simulink model "GPCA_CONFIG"  (Simulink 8.7)
settings: Solver=FixedStepDiscrete  StartTime=0.0  StopTime=10.0  RelTol=1e-3
libraries: simulink x1
settings Model: Creator=bourbouh  LastModifiedBy=bourbouh
settings DataIOCC: LimitDataPoints=off  SaveFormat=Dataset
settings DebuggingCC: UnderspecifiedInitializationDetection=Simplified  MergeDetectMultiDrivingBlocksExec=error
settings HardwareCC: ProdBitPerPointer=64  ProdLargestAtomicFloat=Float  ProdIntDivRoundTo=Zero  ProdEndianess=LittleEndian  ProdWordSize=64  ProdHWDeviceType=Intel->x86-64 (Windows64)
settings ModelReferenceCC: PropagateSignalLabelsOutOfModel=on
settings ConfigComp: CovModelRefEnable=off

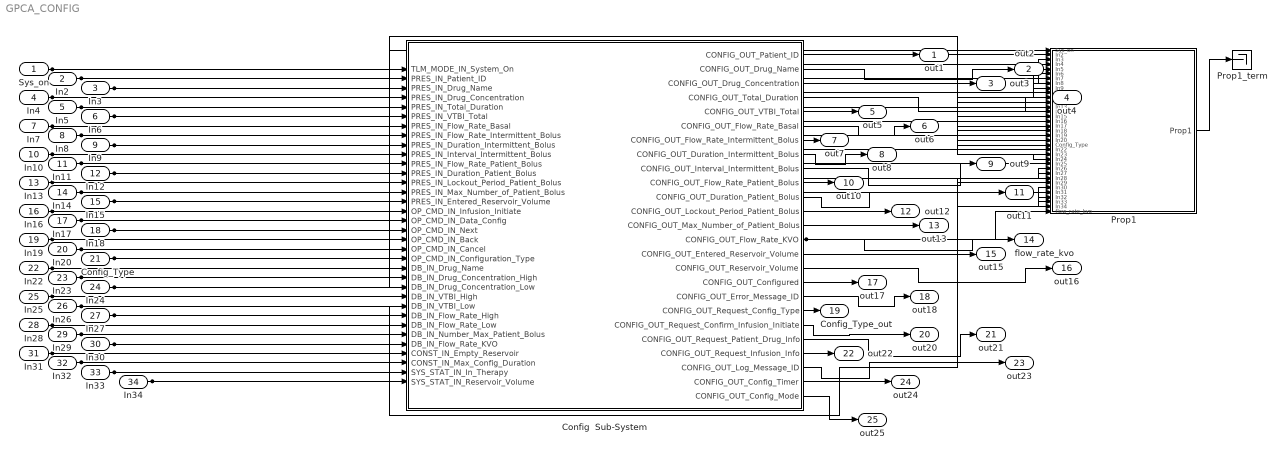
== system GPCA_CONFIG ==
  Sys_on : Inport
  In2 : Inport  Port=2
  In3 : Inport  Port=3
  In4 : Inport  Port=4
  In5 : Inport  Port=5
  In6 : Inport  Port=6
  In7 : Inport  Port=7
  In8 : Inport  Port=8
  In9 : Inport  Port=9
  In10 : Inport  Port=10
  In11 : Inport  Port=11
  In12 : Inport  Port=12
  In13 : Inport  Port=13
  In14 : Inport  Port=14
  In15 : Inport  Port=15
  In16 : Inport  Port=16
  In17 : Inport  Port=17
  In18 : Inport  Port=18
  In19 : Inport  Port=19
  In20 : Inport  Port=20
  Config_Type : Inport  Port=21
  In22 : Inport  Port=22
  In23 : Inport  Port=23
  In24 : Inport  Port=24
  In25 : Inport  Port=25
  In26 : Inport  Port=26
  In27 : Inport  Port=27
  In28 : Inport  Port=28
  In29 : Inport  Port=29
  In30 : Inport  Port=30
  In31 : Inport  Port=31
  In32 : Inport  Port=32
  In33 : Inport  Port=33
  In34 : Inport  Port=34
  Config  Sub-System : Stateflow chart  TreatAsAtomicUnit=on
  Prop1 : Subsystem  TreatAsAtomicUnit=on  mask(Observer){AnnotationType=ensures, ObserverType=[]}
      mask prompts: AnnotationType "Type of annotation (pre/post...)"; ObserverType "Observer type"
      mask help:
      | Set an observer for the system.
      | The annotation type parameter sets the type of observer:
      | - requires : pre-condition
      | - ensures : post-condition
      | - assert : an assertion
      | - observer : the observer computes a special type of properties
      mask TypeOptions AnnotationType: ensures | requires | assert | observer
      mask Callback AnnotationType:
      | paramStr = get_param(gcb, 'MaskValues');
      | if strcmp(paramStr{1}(1),'o')
      | set_param(gcb,'MaskVisibilities',{'on';'on'});
      | paramStr{2} = 'ellipsoid';
      | set_param(gcb,'MaskValues',paramStr);
      | else
      | set_param(gcb,'MaskVisibilities',{'on';'off'});
      | end
      | clear paramStr;
      mask Callback ObserverType:
      | paramStr = get_param(gcb, 'MaskValues');
      | if strcmp(paramStr{1}(1),'o')
      | set_param(gcb,'MaskVisibilities',{'on';'on'});
      | paramStr{2} = 'ellipsoid';
      | set_param(gcb,'MaskValues',paramStr);
      | else
      | set_param(gcb,'MaskVisibilities',{'on';'off'});
      | end
      | clear paramStr;
      mask Display:
      | color('black')
      | text(0.5, 0.5, ['Property: ''' get_param(gcb,'name') ''''], 'horizontalAlignment', 'center');
      | text(0.99, 0.03, '{\bf\fontsize{12}CEX}', 'hor', 'right', 'ver', 'bottom', 'texmode', 'on');
  Prop1_term : Terminator
  out1 : Outport
  out2 : Outport  Port=2
  out3 : Outport  Port=3
  out4 : Outport  Port=4
  out5 : Outport  Port=5
  out6 : Outport  Port=6
  out7 : Outport  Port=7
  out8 : Outport  Port=8
  out9 : Outport  Port=9
  out10 : Outport  Port=10
  out11 : Outport  Port=11
  out12 : Outport  Port=12
  out13 : Outport  Port=13
  flow_rate_kvo : Outport  Port=14
  out15 : Outport  Port=15
  out16 : Outport  Port=16
  out17 : Outport  Port=17
  out18 : Outport  Port=18
  Config_Type_out : Outport  Port=19
  out20 : Outport  Port=20
  out21 : Outport  Port=21
  out22 : Outport  Port=22
  out23 : Outport  Port=23
  out24 : Outport  Port=24
  out25 : Outport  Port=25
  wires:
  Config  Sub-System/2(CONFIG_OUT_Drug_Name) -> out2/1
  Config  Sub-System/3(CONFIG_OUT_Drug_Concentration) -> out3/1
  Config  Sub-System/1(CONFIG_OUT_Patient_ID) -> out1/1
  Config  Sub-System/4(CONFIG_OUT_Total_Duration) -> out4/1
  Config  Sub-System/5(CONFIG_OUT_VTBI_Total) -> out5/1
  Config  Sub-System/6(CONFIG_OUT_Flow_Rate_Basal) -> out6/1
  Config  Sub-System/7(CONFIG_OUT_Flow_Rate_Intermittent_Bolus) -> out7/1
  Config  Sub-System/8(CONFIG_OUT_Duration_Intermittent_Bolus) -> out8/1
  Config  Sub-System/9(CONFIG_OUT_Interval_Intermittent_Bolus) -> out9/1
  Config  Sub-System/12(CONFIG_OUT_Lockout_Period_Patient_Bolus) -> out12/1
  Config  Sub-System/10(CONFIG_OUT_Flow_Rate_Patient_Bolus) -> out10/1
  Config  Sub-System/11(CONFIG_OUT_Duration_Patient_Bolus) -> out11/1
  Config  Sub-System/14(CONFIG_OUT_Flow_Rate_KVO) -> flow_rate_kvo/1, Prop1/35(flow_rate_kvo)
  Config  Sub-System/15(CONFIG_OUT_Entered_Reservoir_Volume) -> out15/1
  Config  Sub-System/13(CONFIG_OUT_Max_Number_of_Patient_Bolus) -> out13/1
  Config  Sub-System/16(CONFIG_OUT_Reservoir_Volume) -> out16/1
  Config  Sub-System/17(CONFIG_OUT_Configured) -> out17/1
  Config  Sub-System/18(CONFIG_OUT_Error_Message_ID) -> out18/1
  Config  Sub-System/20(CONFIG_OUT_Request_Confirm_Infusion_Initiate) -> out20/1
  Config  Sub-System/21(CONFIG_OUT_Request_Patient_Drug_Info) -> out21/1
  Config  Sub-System/24(CONFIG_OUT_Config_Timer) -> out24/1
  Config  Sub-System/22(CONFIG_OUT_Request_Infusion_Info) -> out22/1
  Config  Sub-System/23(CONFIG_OUT_Log_Message_ID) -> out23/1
  Config  Sub-System/19(CONFIG_OUT_Request_Config_Type) -> Config_Type_out/1
  Config  Sub-System/25(CONFIG_OUT_Config_Mode) -> out25/1
  Sys_on/1 -> Config  Sub-System/1(TLM_MODE_IN_System_On), Prop1/1(Sys_on)
  In2/1 -> Config  Sub-System/2(PRES_IN_Patient_ID), Prop1/2(In2)
  In3/1 -> Config  Sub-System/3(PRES_IN_Drug_Name), Prop1/3(In3)
  In4/1 -> Config  Sub-System/4(PRES_IN_Drug_Concentration), Prop1/4(In4)
  In5/1 -> Config  Sub-System/5(PRES_IN_Total_Duration), Prop1/5(In5)
  In6/1 -> Config  Sub-System/6(PRES_IN_VTBI_Total), Prop1/6(In6)
  In7/1 -> Config  Sub-System/7(PRES_IN_Flow_Rate_Basal), Prop1/7(In7)
  In8/1 -> Config  Sub-System/8(PRES_IN_Flow_Rate_Intermittent_Bolus), Prop1/8(In8)
  In9/1 -> Config  Sub-System/9(PRES_IN_Duration_Intermittent_Bolus), Prop1/9(In9)
  In10/1 -> Config  Sub-System/10(PRES_IN_Interval_Intermittent_Bolus), Prop1/10(In10)
  In11/1 -> Config  Sub-System/11(PRES_IN_Flow_Rate_Patient_Bolus), Prop1/11(In11)
  In12/1 -> Config  Sub-System/12(PRES_IN_Duration_Patient_Bolus), Prop1/12(In12)
  In13/1 -> Config  Sub-System/13(PRES_IN_Lockout_Period_Patient_Bolus), Prop1/13(In13)
  In14/1 -> Config  Sub-System/14(PRES_IN_Max_Number_of_Patient_Bolus), Prop1/14(In14)
  In15/1 -> Config  Sub-System/15(PRES_IN_Entered_Reservoir_Volume), Prop1/15(In15)
  In16/1 -> Config  Sub-System/16(OP_CMD_IN_Infusion_Initiate), Prop1/16(In16)
  In17/1 -> Config  Sub-System/17(OP_CMD_IN_Data_Config), Prop1/17(In17)
  In18/1 -> Config  Sub-System/18(OP_CMD_IN_Next), Prop1/18(In18)
  In19/1 -> Config  Sub-System/19(OP_CMD_IN_Back), Prop1/19(In19)
  In20/1 -> Config  Sub-System/20(OP_CMD_IN_Cancel), Prop1/20(In20)
  Config_Type/1 -> Config  Sub-System/21(OP_CMD_IN_Configuration_Type), Prop1/21(Config_Type)
  In22/1 -> Config  Sub-System/22(DB_IN_Drug_Name), Prop1/22(In22)
  In23/1 -> Config  Sub-System/23(DB_IN_Drug_Concentration_High), Prop1/23(In23)
  In24/1 -> Config  Sub-System/24(DB_IN_Drug_Concentration_Low), Prop1/24(In24)
  In25/1 -> Config  Sub-System/25(DB_IN_VTBI_High), Prop1/25(In25)
  In26/1 -> Config  Sub-System/26(DB_IN_VTBI_Low), Prop1/26(In26)
  In27/1 -> Config  Sub-System/27(DB_IN_Flow_Rate_High), Prop1/27(In27)
  In28/1 -> Config  Sub-System/28(DB_IN_Flow_Rate_Low), Prop1/28(In28)
  In29/1 -> Config  Sub-System/29(DB_IN_Number_Max_Patient_Bolus), Prop1/29(In29)
  In30/1 -> Config  Sub-System/30(DB_IN_Flow_Rate_KVO), Prop1/30(In30)
  In31/1 -> Config  Sub-System/31(CONST_IN_Empty_Reservoir), Prop1/31(In31)
  In32/1 -> Config  Sub-System/32(CONST_IN_Max_Config_Duration), Prop1/32(In32)
  In33/1 -> Config  Sub-System/33(SYS_STAT_IN_In_Therapy), Prop1/33(In33)
  In34/1 -> Config  Sub-System/34(SYS_STAT_IN_Reservoir_Volume), Prop1/34(In34)
  Prop1/1(Prop1) -> Prop1_term/1

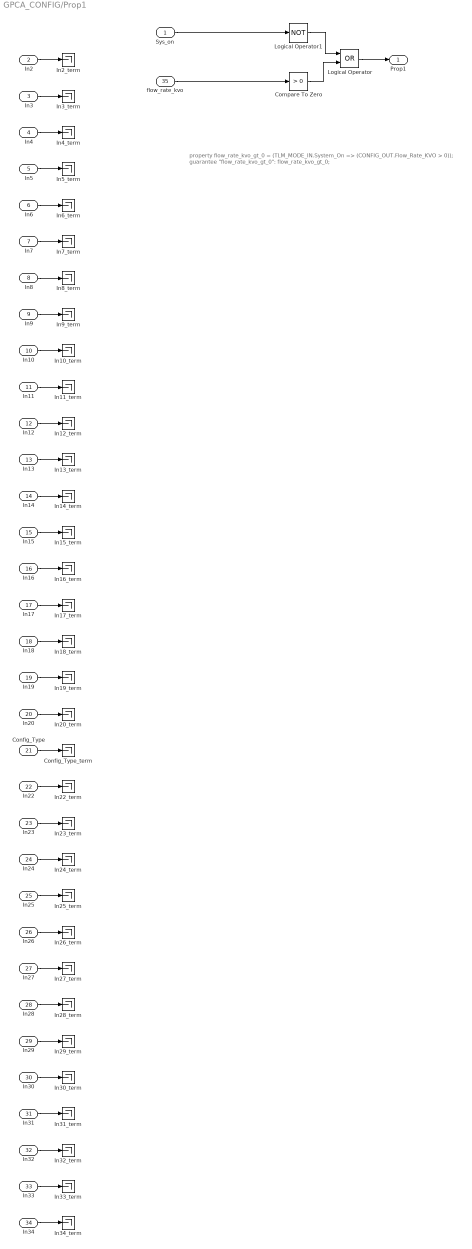
== system GPCA_CONFIG/Prop1 ==
  note: property flow_rate_kvo_gt_0 =
      | (TLM_MODE_IN.System_On => (CONFIG_OUT.Flow_Rate_KVO > 0));
      |
      | guarantee "flow_rate_kvo_gt_0": flow_rate_kvo_gt_0;
  Sys_on : Inport
  In2 : Inport  Port=2
  In3 : Inport  Port=3
  In4 : Inport  Port=4
  In5 : Inport  Port=5
  In6 : Inport  Port=6
  In7 : Inport  Port=7
  In8 : Inport  Port=8
  In9 : Inport  Port=9
  In10 : Inport  Port=10
  In11 : Inport  Port=11
  In12 : Inport  Port=12
  In13 : Inport  Port=13
  In14 : Inport  Port=14
  In15 : Inport  Port=15
  In16 : Inport  Port=16
  In17 : Inport  Port=17
  In18 : Inport  Port=18
  In19 : Inport  Port=19
  In20 : Inport  Port=20
  Config_Type : Inport  Port=21
  In22 : Inport  Port=22
  In23 : Inport  Port=23
  In24 : Inport  Port=24
  In25 : Inport  Port=25
  In26 : Inport  Port=26
  In27 : Inport  Port=27
  In28 : Inport  Port=28
  In29 : Inport  Port=29
  In30 : Inport  Port=30
  In31 : Inport  Port=31
  In32 : Inport  Port=32
  In33 : Inport  Port=33
  In34 : Inport  Port=34
  flow_rate_kvo : Inport  Port=35
  Compare To Zero : simulink/Logic and Bit Operations/Compare To Zero  relop=>  OutDataTypeStr=boolean
  Config_Type_term : Terminator
  In10_term : Terminator
  In11_term : Terminator
  In12_term : Terminator
  In13_term : Terminator
  In14_term : Terminator
  In15_term : Terminator
  In16_term : Terminator
  In17_term : Terminator
  In18_term : Terminator
  In19_term : Terminator
  In20_term : Terminator
  In22_term : Terminator
  In23_term : Terminator
  In24_term : Terminator
  In25_term : Terminator
  In26_term : Terminator
  In27_term : Terminator
  In28_term : Terminator
  In29_term : Terminator
  In2_term : Terminator
  In30_term : Terminator
  In31_term : Terminator
  In32_term : Terminator
  In33_term : Terminator
  In34_term : Terminator
  In3_term : Terminator
  In4_term : Terminator
  In5_term : Terminator
  In6_term : Terminator
  In7_term : Terminator
  In8_term : Terminator
  In9_term : Terminator
  Logical Operator : Logic  Operator=OR  AllPortsSameDT=off  OutDataTypeStr=boolean
  Logical Operator1 : Logic  Operator=NOT  AllPortsSameDT=off  OutDataTypeStr=boolean
  Prop1 : Outport
  wires:
  Sys_on/1 -> Logical Operator1/1
  In2/1 -> In2_term/1
  In3/1 -> In3_term/1
  In4/1 -> In4_term/1
  In5/1 -> In5_term/1
  In6/1 -> In6_term/1
  In7/1 -> In7_term/1
  In8/1 -> In8_term/1
  In9/1 -> In9_term/1
  In10/1 -> In10_term/1
  In11/1 -> In11_term/1
  In12/1 -> In12_term/1
  In13/1 -> In13_term/1
  In14/1 -> In14_term/1
  In15/1 -> In15_term/1
  In16/1 -> In16_term/1
  In17/1 -> In17_term/1
  In18/1 -> In18_term/1
  In19/1 -> In19_term/1
  In20/1 -> In20_term/1
  Config_Type/1 -> Config_Type_term/1
  In22/1 -> In22_term/1
  In23/1 -> In23_term/1
  In24/1 -> In24_term/1
  In25/1 -> In25_term/1
  In26/1 -> In26_term/1
  In27/1 -> In27_term/1
  In28/1 -> In28_term/1
  In29/1 -> In29_term/1
  In30/1 -> In30_term/1
  In31/1 -> In31_term/1
  In32/1 -> In32_term/1
  In33/1 -> In33_term/1
  In34/1 -> In34_term/1
  flow_rate_kvo/1 -> Compare To Zero/1
  Logical Operator/1 -> Prop1/1
  Logical Operator1/1 -> Logical Operator/1
  Compare To Zero/1 -> Logical Operator/2

== stateflow chart Config  Sub-System ==
  state Configuration
    state Prescription_Config
      entry: CONFIG_OUT_Config_Timer++;
      CONFIG_OUT_Reservoir_Volume=SYS_STAT_IN_Reservoir_Volume;
      CONFIG_OUT_Config_Mode=2;
      checkIfPrescriptionAvailable();
      during: CONFIG_OUT_Config_Timer++;
      CONFIG_OUT_Reservoir_Volume=SYS_STAT_IN_Reservoir_Volume;
      checkIfPrescriptionAvailable();
      exit: CONFIG_OUT_Config_Timer++;
      state Patient_Drug_info
        entry: CONFIG_OUT_Config_Mode=3;
        during: CONFIG_OUT_Config_Mode=3;
        exit: CONFIG_OUT_Config_Mode=3;
        state GetParam
          entry:t_PatientID=PRES_IN_Patient_ID;
          t_DrugName=PRES_IN_Drug_Name;
          t_DrugConcentration=PRES_IN_Drug_Concentration;
          t_EnteredReservoirVolume = PRES_IN_Entered_Reservoir_Volume;
          CONFIG_OUT_Request_Patient_Drug_Info=0;
        state DisplayParam
          entry:CONFIG_OUT_Request_Patient_Drug_Info=1;
          validate=0;
        state GetDrugSafeValues
          entry:CONFIG_OUT_Drug_Name=t_DrugName;
          value = CheckDrugName(t_DrugName, DB_IN_Drug_Name);
          during:value = CheckDrugName(t_DrugName, DB_IN_Drug_Name);
        state DisplayErrorMessage
          entry:CONFIG_OUT_Error_Message_ID=5;
        state ValidateParam
          entry:validate= checkPatient_DrugParam(t_DrugConcentration, DB_IN_Drug_Concentration_Low, DB_IN_Drug_Concentration_High, t_EnteredReservoirVolume, CONST_IN_Empty_Reservoir);
          CONFIG_OUT_Request_Patient_Drug_Info=0;
          value=0;
          during:validate= checkPatient_DrugParam(t_DrugConcentration, DB_IN_Drug_Concentration_Low, DB_IN_Drug_Concentration_High, t_EnteredReservoirVolume, CONST_IN_Empty_Reservoir);
          CONFIG_OUT_Request_Patient_Drug_Info=0;
          value=0;
        state v= checkPatient_DrugParam(t_DrugConcentration, DB_IN_Drug_Concentration_Low, DB_IN_Drug_Concentration_High, t_EnteredReservoirVolume, CONST_IN_Empty_Reservoir) [function]
          (default) -> (junction 59) : {v=1;}
          (junction 59) -> (junction 60) [order 1] : [t_DrugConcentration < DB_IN_Drug_Concentration_Low || t_DrugConcentration > DB_IN_Drug_Concentration_High ] {v=0;}
          (junction 59) -> (junction 61) [order 2] : [t_EnteredReservoirVolume < CONST_IN_Empty_Reservoir] {v=0;}
        state y= CheckDrugName(z, DB_IN_Drug_Name) [function]
          (default) -> (junction 68) : {y=1;}
          (junction 68) -> (junction 69) : [z != DB_IN_Drug_Name] {y=0;}
        DisplayParam -> GetParam [order 1] : [OP_CMD_IN_Next == 1]
        (default) -> DisplayParam
        DisplayParam -> ValidateParam [order 2] : [OP_CMD_IN_Next == 1]
        DisplayErrorMessage -> DisplayParam
        GetParam -> GetDrugSafeValues : [OP_CMD_IN_Next == 1]{value=0;}
        GetDrugSafeValues -> DisplayErrorMessage [order 2] : [value==0]
        ValidateParam -> DisplayErrorMessage [order 1] : [validate==0]
        GetDrugSafeValues -> ValidateParam [order 1] : [value==1]
      state SelectType
        entry:CONFIG_OUT_Request_Config_Type=1;
      state Infusion_info
        entry: CONFIG_OUT_Config_Mode=4;
        during: CONFIG_OUT_Config_Mode=4;
        exit: CONFIG_OUT_Config_Mode=4;
        state GetInfusionParam
          entry:t_VTBI_total =PRES_IN_VTBI_Total;
          t_Duration_total =PRES_IN_Total_Duration;
          t_FlowRate_basal =PRES_IN_Flow_Rate_Basal;
          t_FlowRate_sbolus = PRES_IN_Flow_Rate_Intermittent_Bolus;
          t_FlowRate_pbolus =PRES_IN_Flow_Rate_Patient_Bolus;
          t_Duration_sbolus =PRES_IN_Duration_Intermittent_Bolus;
          t_Duration_pbolus =PRES_IN_Duration_Patient_Bolus;
          t_LockOutPeriod_pbolus=PRES_IN_Lockout_Period_Patient_Bolus;
          t_NumberMax_pbolus =PRES_IN_Max_Number_of_Patient_Bolus;
          t_Interval_sbolus =PRES_IN_Interval_Intermittent_Bolus;
          t_FlowRate_kvo =DB_IN_Flow_Rate_KVO;
          CONFIG_OUT_Request_Infusion_Info=0;
        state RequestInfusionParam
          entry :CONFIG_OUT_Request_Infusion_Info=1;
          validate=0;
        state ValidateInfusionParam
          entry: checkInfusionParam();
          during: checkInfusionParam();
        state checkInfusionParam [function]
          (default) -> (junction 79) : {validate=1;}
          (junction 79) -> (junction 78) [order 1] : [t_VTBI_total > DB_IN_VTBI_High || t_VTBI_total < DB_IN_VTBI_Low]{validate=0;}
          (junction 79) -> (junction 80) [order 2] : [t_FlowRate_basal < DB_IN_Flow_Rate_Low || t_FlowRate_basal > DB_IN_Flow_Rate_High]{validate=0;}
          (junction 79) -> (junction 81) [order 3] : [t_FlowRate_sbolus < DB_IN_Flow_Rate_Low || t_FlowRate_sbolus > DB_IN_Flow_Rate_High]{validate=0;}
          (junction 79) -> (junction 82) [order 4] : [t_FlowRate_pbolus< DB_IN_Flow_Rate_Low || t_FlowRate_pbolus > DB_IN_Flow_Rate_High]{validate=0;}
          (junction 79) -> (junction 83) [order 5] : [t_Duration_sbolus  > t_Interval_sbolus]{validate=0;}
          (junction 79) -> (junction 85) [order 7] : [t_FlowRate_pbolus < t_FlowRate_basal || t_FlowRate_sbolus < t_FlowRate_basal ]{validate=0;}
          (junction 79) -> (junction 84) [order 6] : [t_NumberMax_pbolus >  DB_IN_Number_Max_Patient_Bolus]{validate=0;}
        RequestInfusionParam -> GetInfusionParam [order 1] : [OP_CMD_IN_Next == 1]
        (default) -> RequestInfusionParam
        ValidateInfusionParam -> RequestInfusionParam [order 1] : [validate==0]
        RequestInfusionParam -> ValidateInfusionParam [order 2] : [OP_CMD_IN_Next == 1]
        GetInfusionParam -> ValidateInfusionParam : [OP_CMD_IN_Next == 1]
      state ConfirmInfusionInitation
        entry:CONFIG_OUT_Request_Confirm_Infusion_Initiate = 1;
        during: CONFIG_OUT_Request_Confirm_Infusion_Initiate = 1;
      (default) -> SelectType
      SelectType -> (junction 34) : [OP_CMD_IN_Configuration_Type>0] {CONFIG_OUT_Request_Config_Type=0;Selected_Configuration_Type=OP_CMD_IN_Configuration_Type;copyCurrentValuesToTemp();}
      (junction 34) -> Patient_Drug_info [order 2]
      (junction 34) -> Infusion_info [order 1] : [SYS_STAT_IN_In_Therapy]
      Infusion_info -> Patient_Drug_info : [OP_CMD_IN_Back && !SYS_STAT_IN_In_Therapy]
      ValidateParam -> Infusion_info [order 2] : [validate==1]
      ValidateInfusionParam -> ConfirmInfusionInitation [order 2] : [validate==1]
    state MAIN
      entry: CONFIG_OUT_Config_Mode=1;
      CONFIG_OUT_Config_Timer=0;
      setReservoirVolume();
      checkIfPrescriptionAvailable();
      during: CONFIG_OUT_Config_Mode=1;
      CONFIG_OUT_Config_Timer=0;
      setReservoirVolume();
      checkIfPrescriptionAvailable();
      exit: CONFIG_OUT_Config_Mode=1;
      CONFIG_OUT_Config_Timer=0;
      setReservoirVolume();
      checkIfPrescriptionAvailable();
    state copyCurrentValuesToTemp [function]
      (default) -> (junction 94) : {t_PatientID= CONFIG_OUT_Patient_ID;
          | t_DrugName=CONFIG_OUT_Drug_Name;
          | t_DrugConcentration= CONFIG_OUT_Drug_Concentration;
          | t_EnteredReservoirVolume=CONFIG_OUT_Entered_Reservoir_Volume;
          | t_VTBI_total=CONFIG_OUT_VTBI_Total;
          | t_Duration_total=CONFIG_OUT_Total_Duration;
          | t_FlowRate_basal=CONFIG_OUT_Flow_Rate_Basal;
          | t_FlowRate_sbolus=CONFIG_OUT_Flow_Rate_Intermittent_Bolus;
          | t_FlowRate_pbolus=CONFIG_OUT_Flow_Rate_Patient_Bolus;
          | t_FlowRate_kvo=CONFIG_OUT_Flow_Rate_KVO;
          | t_Duration_sbolus=CONFIG_OUT_Duration_Intermittent_Bolus;
          | t_Duration_pbolus=CONFIG_OUT_Duration_Patient_Bolus;
          | t_LockOutPeriod_pbolus=CONFIG_OUT_Lockout_Period_Patient_Bolus;
          | t_NumberMax_pbolus=CONFIG_OUT_Max_Number_of_Patient_Bolus;
          | t_Interval_sbolus=CONFIG_OUT_Interval_Intermittent_Bolus;
          | t_EnteredReservoirVolume=CONFIG_OUT_Entered_Reservoir_Volume;}
    state saveConfigValues [function]
      (default) -> (junction 96) : {CONFIG_OUT_Patient_ID=t_PatientID;
          | CONFIG_OUT_Drug_Name=t_DrugName;
          | CONFIG_OUT_Drug_Concentration=t_DrugConcentration;
          | CONFIG_OUT_Entered_Reservoir_Volume = t_EnteredReservoirVolume;
          | CONFIG_OUT_VTBI_Total =t_VTBI_total;
          | CONFIG_OUT_Total_Duration =t_Duration_total;
          | CONFIG_OUT_Flow_Rate_Basal =t_FlowRate_basal;
          | CONFIG_OUT_Flow_Rate_Intermittent_Bolus = t_FlowRate_sbolus;
          | CONFIG_OUT_Flow_Rate_Patient_Bolus =t_FlowRate_pbolus;
          | CONFIG_OUT_Flow_Rate_KVO =t_FlowRate_kvo;
          | CONFIG_OUT_Duration_Intermittent_Bolus =t_Duration_sbolus;
          | CONFIG_OUT_Duration_Patient_Bolus =t_Duration_pbolus;
          | CONFIG_OUT_Lockout_Period_Patient_Bolus =t_LockOutPeriod_pbolus;
          | CONFIG_OUT_Max_Number_of_Patient_Bolus =t_NumberMax_pbolus;
          | CONFIG_OUT_Interval_Intermittent_Bolus =t_Interval_sbolus;
          | CONFIG_OUT_Reservoir_Volume=CONFIG_OUT_Entered_Reservoir_Volume;
          | CONFIG_OUT_Configured=Selected_Configuration_Type;
          | New_Configuration=1;
          | /*cancelConfigValues();*/
          | /*comment it because it is in the same level*/
          | /*Try to call cancelConfigValues every time you call the current function*/
          | writeLog(1);}
    state cancelConfigValues [function]
      (default) -> (junction 98) : {t_PatientID=0;
          | t_DrugName=0;
          | t_DrugConcentration=0;
          | t_EnteredReservoirVolume =0;
          | t_VTBI_total =0 ;
          | t_Duration_total =0 ;
          | t_FlowRate_basal =0 ;
          | t_FlowRate_sbolus =0 ;
          | t_FlowRate_pbolus =0 ;
          | t_FlowRate_kvo =0 ;
          | t_Duration_sbolus =0 ;
          | t_Duration_pbolus =0 ;
          | t_LockOutPeriod_pbolus =0 ;
          | t_NumberMax_pbolus =0 ;
          | t_Interval_sbolus =0 ;
          | writeLog(2);}
    state checkIfPrescriptionAvailable [function]
      (default) -> (junction 100)
      (junction 100) -> (junction 101) [order 1] : [!New_Configuration]
      (junction 100) -> (junction 104) [order 2] : {New_Configuration=0;}
      (junction 101) -> (junction 102) [order 1] : [(CONFIG_OUT_Patient_ID > 0) && (CONFIG_OUT_Drug_Name>0) && (CONFIG_OUT_Drug_Concentration >0) && (CONFIG_OUT_VTBI_Total >0 ) && (CONFIG_OUT_Total_Duration >0 ) && (CONFIG_OUT_Flow_Rate_Basal > 0)] {CONFIG_OUT_Configured =3;}
      (junction 101) -> (junction 103) [order 2] : {CONFIG_OUT_Configured =0;}
    state setReservoirVolume [function]
      (default) -> (junction 110) : [!New_Configuration]{CONFIG_OUT_Reservoir_Volume=SYS_STAT_IN_Reservoir_Volume;}
    (default) -> MAIN
    MAIN -> Prescription_Config : [OP_CMD_IN_Data_Config || (OP_CMD_IN_Infusion_Initiate && CONFIG_OUT_Configured ==0 ) ]
    Prescription_Config -> MAIN : [(CONFIG_OUT_Config_Timer > Step_Scaling_Factor(CONST_IN_Max_Config_Duration,step_size)) || OP_CMD_IN_Cancel]{cancelConfigValues();}
    ConfirmInfusionInitation -> MAIN : [OP_CMD_IN_Infusion_Initiate]{CONFIG_OUT_Request_Confirm_Infusion_Initiate=0;saveConfigValues();cancelConfigValues();}
  state NOT_ON
  state writeLog(logEvent) [function]
    (default) -> (junction 113) : {CONFIG_OUT_Log_Message_ID=logEvent;}
  state returnVal = Step_Scaling_Factor(inputVal,step_size) [function]
    (default) -> (junction 118) : {returnVal= inputVal/step_size;}
  note: step scaling factor returns the scaled time depending upon the step size.
      | If counter has to timeout after 100 seconds and if the step size is 0.1 second
      | the new timeout value = 100/0.1 = 1000 steps.
      | default will be one step = 1 second.
  (default) -> Configuration [order 1] : [TLM_MODE_IN_System_On]
  (default) -> NOT_ON [order 2]
  NOT_ON -> Configuration : [TLM_MODE_IN_System_On]
  Configuration -> NOT_ON : [!TLM_MODE_IN_System_On]
  data: v function_output uint8; t_DrugConcentration function_input uint8; DB_IN_Drug_Concentration_Low function_input uint8; DB_IN_Drug_Concentration_High function_input uint8; t_EnteredReservoirVolume function_input uint8; CONST_IN_Empty_Reservoir function_input uint8; y function_output uint8; z function_input uint8; DB_IN_Drug_Name function_input uint8; logEvent function_input uint8; inputVal function_input double; returnVal function_output double; step_size function_input double; TLM_MODE_IN_System_On input boolean; CONFIG_OUT_Patient_ID output uint8; PRES_IN_Patient_ID input uint8; PRES_IN_Drug_Name input uint8; PRES_IN_Drug_Concentration input uint8; PRES_IN_Total_Duration input uint8; PRES_IN_VTBI_Total input uint8; PRES_IN_Flow_Rate_Basal input uint8; PRES_IN_Flow_Rate_Intermittent_Bolus input uint8; PRES_IN_Duration_Intermittent_Bolus input uint8; PRES_IN_Interval_Intermittent_Bolus input uint8; PRES_IN_Flow_Rate_Patient_Bolus input uint8; PRES_IN_Duration_Patient_Bolus input uint8; PRES_IN_Lockout_Period_Patient_Bolus input uint8; PRES_IN_Max_Number_of_Patient_Bolus input uint8; PRES_IN_Entered_Reservoir_Volume input uint8; OP_CMD_IN_Infusion_Initiate input boolean; OP_CMD_IN_Data_Config input boolean; OP_CMD_IN_Next input boolean; OP_CMD_IN_Back input boolean; OP_CMD_IN_Cancel input boolean; OP_CMD_IN_Configuration_Type input uint8; DB_IN_Drug_Name input uint8; DB_IN_Drug_Concentration_High input uint8; DB_IN_Drug_Concentration_Low input uint8; DB_IN_VTBI_High input uint8; DB_IN_VTBI_Low input uint8; DB_IN_Flow_Rate_High input uint8; DB_IN_Flow_Rate_Low input uint8; DB_IN_Number_Max_Patient_Bolus input uint8; CONFIG_OUT_Drug_Name output uint8; CONFIG_OUT_Drug_Concentration output uint8; CONFIG_OUT_Total_Duration output uint8; CONFIG_OUT_VTBI_Total output uint8; CONFIG_OUT_Flow_Rate_Basal output uint8; CONFIG_OUT_Flow_Rate_Intermittent_Bolus output uint8; CONFIG_OUT_Duration_Intermittent_Bolus output uint8; CONFIG_OUT_Interval_Intermittent_Bolus output uint8; CONFIG_OUT_Flow_Rate_Patient_Bolus output uint8; CONFIG_OUT_Duration_Patient_Bolus output uint8; CONFIG_OUT_Lockout_Period_Patient_Bolus output uint8; CONFIG_OUT_Max_Number_of_Patient_Bolus output uint8; CONFIG_OUT_Flow_Rate_KVO output uint8; DB_IN_Flow_Rate_KVO input uint8; CONFIG_OUT_Entered_Reservoir_Volume output uint8; CONFIG_OUT_Reservoir_Volume output uint8; CONFIG_OUT_Configured output uint8; CONST_IN_Empty_Reservoir input uint8; CONST_IN_Max_Config_Duration input double; CONFIG_OUT_Error_Message_ID output uint8; CONFIG_OUT_Request_Config_Type output boolean; CONFIG_OUT_Request_Confirm_Infusion_Initiate output boolean; CONFIG_OUT_Request_Patient_Drug_Info output boolean; CONFIG_OUT_Request_Infusion_Info output boolean; t_DrugConcentration local uint8; t_DrugName local uint8; t_Duration_pbolus local uint8; t_Duration_sbolus local uint8; t_Duration_total local uint8; t_FlowRate_basal local uint8; t_FlowRate_kvo local uint8; t_FlowRate_pbolus local uint8; t_FlowRate_sbolus local uint8; t_Interval_sbolus local uint8; t_LockOutPeriod_pbolus local uint8; t_NumberMax_pbolus local uint8; t_PatientID local uint8; t_EnteredReservoirVolume local uint8; t_VTBI_total local uint8; validate local uint8; value local uint8; SYS_STAT_IN_In_Therapy input boolean; CONFIG_OUT_Log_Message_ID output uint8; CONFIG_OUT_Config_Timer output double; SYS_STAT_IN_Reservoir_Volume input uint8; step_size parameter double; CONFIG_OUT_Config_Mode output uint8; New_Configuration local boolean; Selected_Configuration_Type local uint8
